simulink model "LQR-2"  (R2018a)
settings: Solver=VariableStepAuto  StartTime=0.0  StopTime=100  RelTol=1e-3
libraries: simulink x1
settings Model: Creator=86153  LastModifiedBy=86153

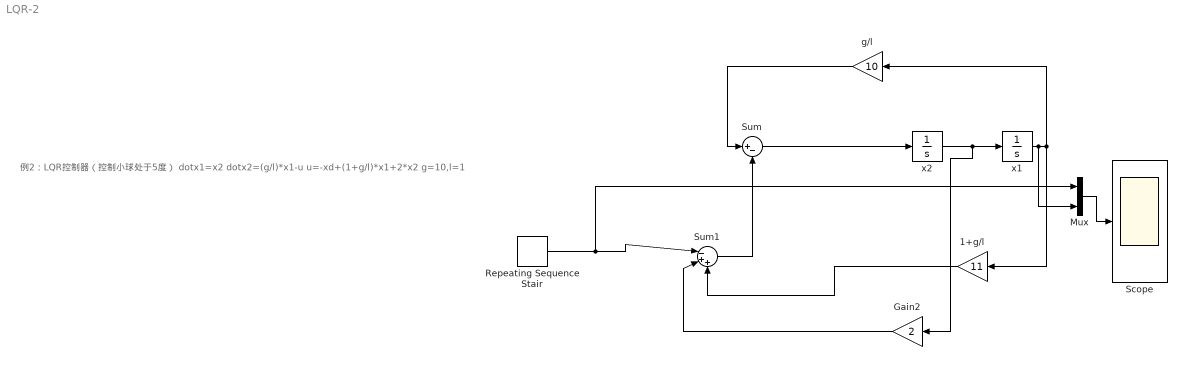
== system LQR-2 ==
  note: 例2：LQR控制器（控制小球处于5度）
      | dotx1=x2
      | dotx2=(g/l)*x1-u
      | u=-xd+(1+g/l)*x1+2*x2
      | g=10,l=1
  1+g/l : Gain  Gain=11
  Gain2 : Gain  Gain=2
  Mux : Mux  Inputs=2
  Repeating Sequence Stair : simulink/Sources/Repeating Sequence Stair  OutValues=[3 1 4 2 1].'  tsamp=20  OutMin=[]  OutMax=[]  OutDataTypeStr=double  OutputDataTypeScalingMode=double  OutDataType=fixdt(0,8)  ConRadixGroup=Best Precision: Vector-wise  OutScaling=2^-12
  Scope : Scope
  Sum : Sum  Inputs=|+-
  Sum1 : Sum  Inputs=|-++
  g/l : Gain  Gain=10
  x1 : Integrator
  x2 : Integrator
  wires:
  x2/1 -> Gain2/1, x1/1
  x1/1 -> Mux/2, 1+g/l/1, g/l/1
  g/l/1 -> Sum/1
  Sum/1 -> x2/1
  Repeating Sequence Stair/1 -> Mux/1, Sum1/1
  Gain2/1 -> Sum1/2
  1+g/l/1 -> Sum1/3
  Sum1/1 -> Sum/2
  Mux/1 -> Scope/1
